simulink model "three_phase_hw_lr"  (Simulink 6.1)
settings: Solver=ode23tb  StartTime=0.0  StopTime=0.1499  MaxStep=1e-4  RelTol=1e-3  AbsTol=.01
libraries: powerlib x12
settings Model: LastModifiedBy=ThinkPad
settings DebuggingCC: SolverPrmCheckMsg=warning

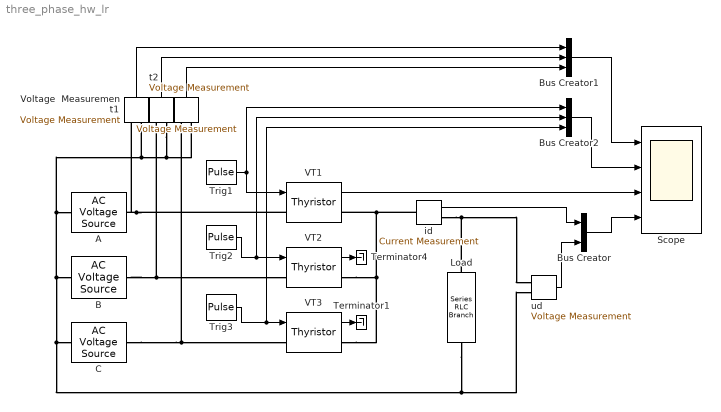
== system three_phase_hw_lr ==
  "   " : powerlib/Measurements/Voltage Measurement  Orientation=up  PhasorSimulation=off  OutputType=Complex  PSBequivalent=0
  A : powerlib/Electrical Sources/AC Voltage Source  Amplitude=100  Phase=30  Frequency=50  SampleTime=0  Measurements=None
  B : powerlib/Electrical Sources/AC Voltage Source  Amplitude=100  Phase=-90  Frequency=50  SampleTime=0  Measurements=None
  Bus Creator : BusCreator  DialogController=Simulink.DDGSource_Bus  Inputs=2
  Bus Creator1 : BusCreator  DialogController=Simulink.DDGSource_Bus  Inputs=3
  Bus Creator2 : BusCreator  DialogController=Simulink.DDGSource_Bus  Inputs=3
  C : powerlib/Electrical Sources/AC Voltage Source  Amplitude=100  Phase=-210  Frequency=50  SampleTime=0  Measurements=None
  Load : powerlib/Elements/Series RLC Branch  Orientation=down  PhysicalDomain=powersysdomain  SubClassName=unknown  LeftPortType=p1  RightPortType=p1  LConnTagsString=__new0  RConnTagsString=__new0  Resistance=1  Inductance=0.05  Capacitance=inf  Measurements=None
  Scope : Scope  NumInputPorts=4
      settings: TimeRange=0.05  YMin=-100~-50~-200~-100  YMax=100~50~200~100  Decimation=5  SampleInput=on  SampleTime=1e-4
  Terminator1 : Terminator
  Terminator4 : Terminator
  Trig1 : DiscretePulseGenerator  PulseType=Time based  Amplitude=10  Period=0.02  PulseWidth=5  PhaseDelay=0.00333
  Trig2 : DiscretePulseGenerator  PulseType=Time based  Amplitude=10  Period=0.02  PulseWidth=5  PhaseDelay=0.01
  Trig3 : DiscretePulseGenerator  PulseType=Time based  Amplitude=10  Period=0.02  PulseWidth=5  PhaseDelay=0.01667
  VT1 : powerlib/Power Electronics/Thyristor  Ron=0.01  Lon=0  Vf=0.8  IC=0  Rs=1000  Cs=100e-9  Measurements=on
  VT2 : powerlib/Power Electronics/Thyristor  Ron=0.01  Lon=0  Vf=0.8  IC=0  Rs=1000  Cs=100e-9  Measurements=on
  VT3 : powerlib/Power Electronics/Thyristor  Ron=0.01  Lon=0  Vf=0.8  IC=0  Rs=1000  Cs=100e-9  Measurements=on
  Voltage  Measurement1 : powerlib/Measurements/Voltage Measurement  Orientation=up  PhasorSimulation=off  OutputType=Complex  PSBequivalent=0
  id : powerlib/Measurements/Current Measurement  PhasorSimulation=off  OutputType=Complex  PSBequivalent=0
  t2 : powerlib/Measurements/Voltage Measurement  Orientation=up  PhasorSimulation=off  OutputType=Complex  PSBequivalent=0
  ud : powerlib/Measurements/Voltage Measurement  PhasorSimulation=off  OutputType=Complex  PSBequivalent=0
  wires:
  VT1/1 -> Scope/3
  ud/1 -> Bus Creator/2
  Bus Creator/1 -> Scope/4
  id/1 -> Bus Creator/1
  Trig3/1 -> VT3/1, Bus Creator2/3
  Bus Creator1/1 -> Scope/1
  Voltage  Measurement1/1 -> Bus Creator1/1
  Trig2/1 -> VT2/1, Bus Creator2/2
  Bus Creator2/1 -> Scope/2
  Trig1/1 -> VT1/1, Bus Creator2/1
  t2/1 -> Bus Creator1/2
  "   "/1 -> Bus Creator1/3
  VT3/1 -> Terminator1/1
  VT2/1 -> Terminator4/1
  connections:
  id/RConn1 -- Load/LConn1 -- ud/LConn1
  VT3/RConn1 -- id/LConn1 -- VT1/RConn1 -- VT2/RConn1
  B/LConn1 -- t2/LConn2 -- "   "/LConn2 -- Voltage  Measurement1/LConn2 -- A/LConn1 -- Load/RConn1 -- ud/LConn2 -- C/LConn1
  A/RConn1 -- VT1/LConn1 -- Voltage  Measurement1/LConn1
  t2/LConn1 -- B/RConn1 -- VT2/LConn1
  C/RConn1 -- VT3/LConn1 -- "   "/LConn1
